simulink model "Comparing_thermoconduction_vs_heat_transfer_coeff"  (R2015a)
settings: Solver=ode45  StartTime=0.0  StopTime=100  MaxStep=0.1  RelTol=1e-3
libraries: fl_lib x12, nesl_utility x4
settings Model: Creator=Oleg  LastModifiedBy=Oleg

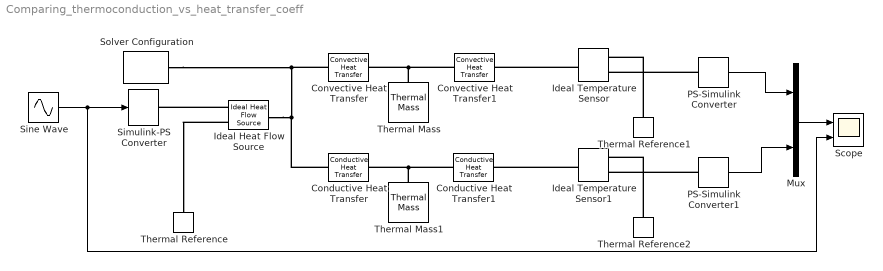
== system Comparing_thermoconduction_vs_heat_transfer_coeff ==
  Conductive Heat Transfer : fl_lib/Thermal/Thermal Elements/Conductive Heat Transfer  area=2 m^2  thickness=2 m  th_cond=60 W/(m*K)  Q_specify=off  Q_priority=High  Q=0 J/s  T_specify=off  T_priority=High  T=0 K
  Conductive Heat Transfer1 : fl_lib/Thermal/Thermal Elements/Conductive Heat Transfer  area=2 m^2  thickness=2 m  th_cond=60 W/(m*K)  Q_specify=off  Q_priority=High  Q=0 J/s  T_specify=off  T_priority=High  T=0 K
  Convective Heat Transfer : fl_lib/Thermal/Thermal Elements/Convective Heat Transfer  area=2 m^2  heat_tr_coeff=30 W/(m^2 * K)  Q_specify=off  Q_priority=High  Q=0 J/s  T_specify=off  T_priority=High  T=0 K
  Convective Heat Transfer1 : fl_lib/Thermal/Thermal Elements/Convective Heat Transfer  area=2 m^2  heat_tr_coeff=30 W/(m^2 * K)  Q_specify=off  Q_priority=High  Q=0 J/s  T_specify=off  T_priority=High  T=0 K
  Ideal Heat Flow Source : fl_lib/Thermal/Thermal Sources/Ideal Heat Flow Source
  Ideal Temperature Sensor : fl_lib/Thermal/Thermal Sensors/Ideal Temperature Sensor
  Ideal Temperature Sensor1 : fl_lib/Thermal/Thermal Sensors/Ideal Temperature Sensor
  Mux : Mux  Inputs=2
  PS-Simulink Converter : nesl_utility/PS-Simulink Converter  PhysicalDomain=network_engine_domain  SubClassName=ps_output  LeftPortType=input  RightPortType=output  PseudoPeriodic=off  Frequencies=[]  Unit=1  AffineConversion=off
  PS-Simulink Converter1 : nesl_utility/PS-Simulink Converter  PhysicalDomain=network_engine_domain  SubClassName=ps_output  LeftPortType=input  RightPortType=output  PseudoPeriodic=off  Frequencies=[]  Unit=1  AffineConversion=off
  Scope : Scope  NumInputPorts=2
      settings: YMin=-5~-5  YMax=5~5
  Simulink-PS Converter : nesl_utility/Simulink-PS Converter  PhysicalDomain=network_engine_domain  SubClassName=ps_input  LeftPortType=input  RightPortType=output  PseudoPeriodic=off  Frequencies=[]  NoiseDistribution=none  NoiseParameters=[]  Unit=1  AffineConversion=off  InputFiltering=off  SimscapeFilterOrder=1  InputFilterTimeConstant=0.001  UdotUserProvided=1
  Sine Wave : Sin  SampleTime=0
  Solver Configuration : nesl_utility/Solver Configuration  PhysicalDomain=network_engine_domain  SubClassName=solver  LeftPortType=input  RightPortType=generic  Accelerate=off  Tones=[]  Harmonics=[]  SimulateNoise=off  Profile=off  UseLocalSampling=off  EnableSwitchedLinearOptims=on  FrequencyDomain=off  UseCCode=off  RelTol=0.001  AbsTol=1e-06  MinStep=1e-09  ToWorkspace=off  RevertToSquareIcSolve=off  NumHomotopyIterations=100  DoDC=off  ResidualTolerance=1e-09  UseLocalSolver=off  LocalSolverChoice=NE_BACKWARD_EULER_ADVANCER  LocalSolverSampleTime=0.001  DoFixedCost=off  MaxNonlinIter=3  MaxModeIter=2  LinearAlgebra=Sparse  DelaysMemoryBudget=1024  AutomaticFiltering=on  FilteringTimeConstant=0.001
  Thermal Mass : fl_lib/Thermal/Thermal Elements/Thermal Mass  mass=1 kg  sp_heat=447 J/kg/K  Q_specify=off  Q_priority=High  Q=0 J/s  T_specify=off  T_priority=High  T=300 K
  Thermal Mass1 : fl_lib/Thermal/Thermal Elements/Thermal Mass  mass=1 kg  sp_heat=447 J/kg/K  Q_specify=off  Q_priority=High  Q=0 J/s  T_specify=off  T_priority=High  T=300 K
  Thermal Reference : fl_lib/Thermal/Thermal Elements/Thermal Reference
  Thermal Reference1 : fl_lib/Thermal/Thermal Elements/Thermal Reference
  Thermal Reference2 : fl_lib/Thermal/Thermal Elements/Thermal Reference
  wires:
  Sine Wave/1 -> Scope/2, Simulink-PS Converter/1
  PS-Simulink Converter/1 -> Mux/1
  PS-Simulink Converter1/1 -> Mux/2
  Mux/1 -> Scope/1
  connections:
  Ideal Heat Flow Source/RConn1 -- Simulink-PS Converter/RConn1
  Ideal Heat Flow Source/RConn2 -- Thermal Reference/LConn1
  Convective Heat Transfer/LConn1 -- Solver Configuration/RConn1 -- Ideal Heat Flow Source/LConn1 -- Conductive Heat Transfer/LConn1
  Thermal Mass/LConn1 -- Convective Heat Transfer1/LConn1 -- Convective Heat Transfer/RConn1
  Thermal Mass1/LConn1 -- Conductive Heat Transfer1/LConn1 -- Conductive Heat Transfer/RConn1
  PS-Simulink Converter/LConn1 -- Ideal Temperature Sensor/RConn2
  Thermal Reference1/LConn1 -- Ideal Temperature Sensor/RConn1
  PS-Simulink Converter1/LConn1 -- Ideal Temperature Sensor1/RConn2
  Thermal Reference2/LConn1 -- Ideal Temperature Sensor1/RConn1
  Ideal Temperature Sensor1/LConn1 -- Conductive Heat Transfer1/RConn1
  Ideal Temperature Sensor/LConn1 -- Convective Heat Transfer1/RConn1
